simulink model "suspenstionOptimizer"  (R2025a)
settings: Solver=VariableStepAuto  StartTime=0.0  StopTime=250.0  RelTol=1e-3
undefined symbols (not defined in the file or in its folder): cs, ks, mass_payload, mass_robot
libraries: checkpacklib x1
settings Model: DataDictionary=Constants.sldd  Creator=levirogalla  LastModifiedBy=levirogalla

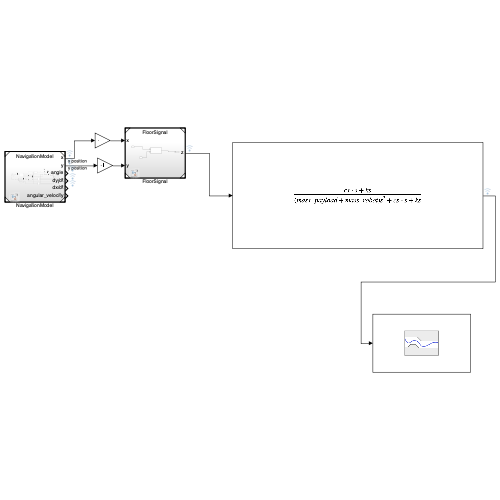
[thumbnail: Simulink's stored preview of the top-level diagram]
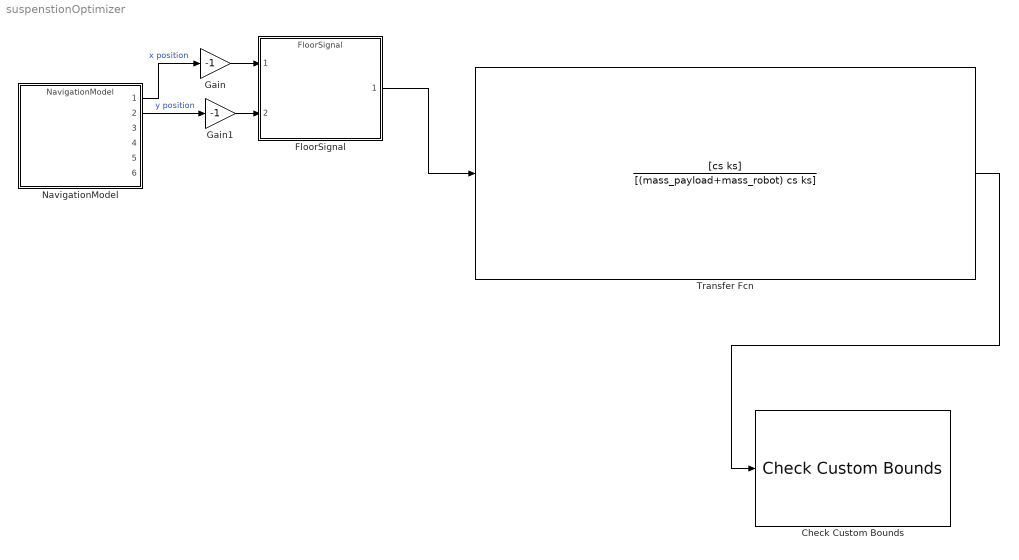
== system suspenstionOptimizer ==
  Check Custom Bounds : checkpacklib/Check Custom Bounds  InstantiateOnLoad=on  enabled=on  stopWhenAssertionFail=off  export=off  ViewDlgPos=[]  OpenViewOnLoad=off  LaunchViewOnOpen=off  TimeUnits=seconds  EnableUpperBound=on  UpperBoundTimes=[0 20]  UpperBoundAmplitudes=[0.005 0.005];  EnableLowerBound=on  LowerBoundTimes=[0 20]  LowerBoundAmplitudes=[-0.005 -0.005]
      settings: LibrarySourceBlock=sdolib/Model Verification/Check Custom Bounds
  FloorSignal : ModelReference  ModelNameDialog=FloorSignal.slx  SimulationMode=Normal  ModelReferenceVersion=1.9
  Gain : Gain  Gain=-1
  Gain1 : Gain  Gain=-1
  NavigationModel : ModelReference  ModelNameDialog=NavigationModel.slx  SimulationMode=Normal  ModelReferenceVersion=1.99
  Transfer Fcn : TransferFcn  Numerator=[cs ks]  Denominator=[(mass_payload+mass_robot) cs ks]
  wires:
  NavigationModel/1 -> Gain/1  "x position"
  NavigationModel/2 -> Gain1/1  "y position"
  Gain/1 -> FloorSignal/1
  Gain1/1 -> FloorSignal/2
  FloorSignal/1 -> Transfer Fcn/1
  Transfer Fcn/1 -> Check Custom Bounds/1
